simulink model "LRMate200Experimentor_Servo"  (R2015b)
settings: Solver=FixedStepDiscrete  StartTime=0.0  StopTime=10.0  FixedStep=si.tsv  RelTol=1e-3
model workspace (MATLAB code in the model file):
  | rsi = evalin('base', 'si.ri{1}');
undefined symbols (not defined in the file or in its folder): DiscIntNeverNeededParam, si
libraries: simulink x7
settings Model: ParameterArgumentNames=rsi  Creator=rluser  LastModifiedBy=Chin
settings SolverCC: EnableConcurrentExecution=on
settings DataIOCC: SaveFormat=Array
settings OptimizationCC: BlockReduction=off  OptimizeBlockIOStorage=off  BufferReuse=off  GlobalBufferReuse=off  ExpressionFolding=off  LocalBlockOutputs=off
settings DebuggingCC: SolverPrmCheckMsg=warning
settings HardwareCC: ProdBitPerPointer=32  ProdLargestAtomicFloat=None  ProdWordSize=32  ProdLongLongMode=on  ProdHWDeviceType=Generic->32-bit x86 compatible
settings RTWCC: SystemTargetFile=slrt.tlc  TemplateMakefile=slrt_default_tmf  Description=Simulink Real-Time  RTWCompilerOptimization=on
settings CodeAppCC: MaxIdLength=120
settings SimulinkRealTimeCC: GeneratePreprocessorConditionals=Disable all
settings ConfigComp: CovModelRefEnable=Off  CovSFcnEnable=off

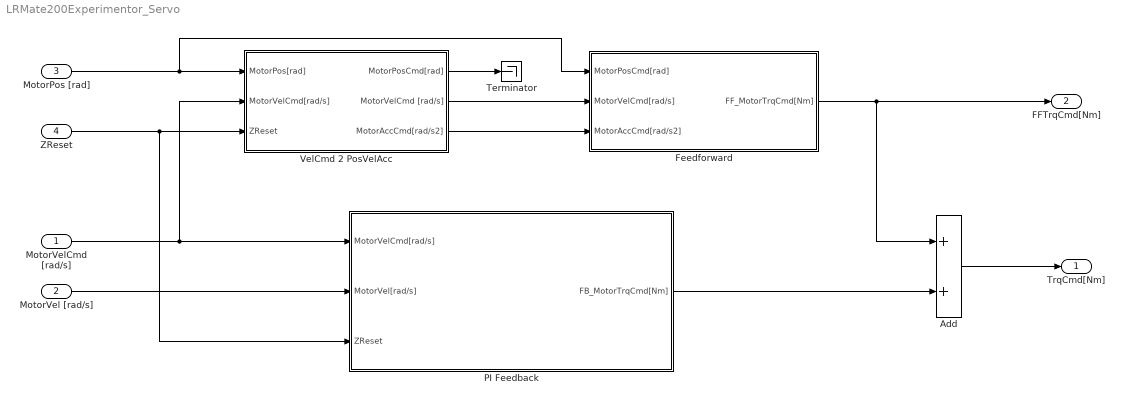
== system LRMate200Experimentor_Servo ==
  MotorVelCmd [rad/s] : Inport  PortDimensions=6
  MotorVel [rad/s] : Inport  Port=2  PortDimensions=6
  MotorPos [rad] : Inport  Port=3  PortDimensions=6
  ZReset : Inport  Port=4  OutDataTypeStr=boolean
  Add : Sum
  Feedforward : Subsystem
  PI Feedback : Subsystem
  Terminator : Terminator
  VelCmd 2 PosVelAcc : Subsystem
  TrqCmd[Nm] : Outport
  FFTrqCmd[Nm] : Outport  Port=2
  wires:
  MotorVel [rad/s]/1 -> PI Feedback/2(MotorVel[rad/s])
  MotorVelCmd [rad/s]/1 -> VelCmd 2 PosVelAcc/2(MotorVelCmd[rad/s]), PI Feedback/1(MotorVelCmd[rad/s])
  Add/1 -> TrqCmd[Nm]/1
  MotorPos [rad]/1 -> Feedforward/1(MotorPosCmd[rad]), VelCmd 2 PosVelAcc/1(MotorPos[rad])
  VelCmd 2 PosVelAcc/2(MotorVelCmd [rad/s]) -> Feedforward/2(MotorVelCmd[rad/s])
  VelCmd 2 PosVelAcc/3(MotorAccCmd[rad/s2]) -> Feedforward/3(MotorAccCmd[rad/s2])
  VelCmd 2 PosVelAcc/1(MotorPosCmd[rad]) -> Terminator/1
  ZReset/1 -> PI Feedback/3(ZReset), VelCmd 2 PosVelAcc/3(ZReset)
  PI Feedback/1(FB_MotorTrqCmd[Nm]) -> Add/2
  Feedforward/1(FF_MotorTrqCmd[Nm]) -> FFTrqCmd[Nm]/1, Add/1

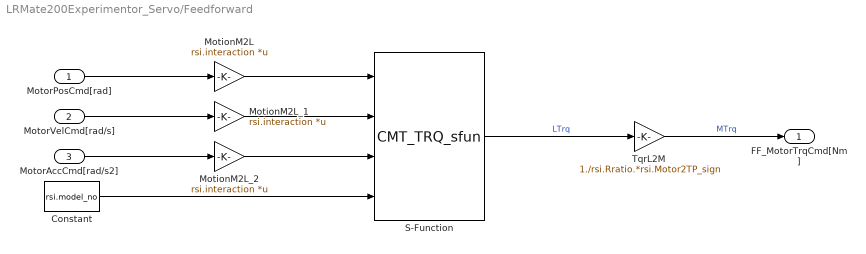
== system LRMate200Experimentor_Servo/Feedforward ==
  MotorPosCmd[rad] : Inport
  MotorVelCmd[rad/s] : Inport  Port=2
  MotorAccCmd[rad/s2] : Inport  Port=3
  Constant : Constant  Value=rsi.model_no
  MotionM2L : Gain  Gain=rsi.interaction  Multiplication=Matrix(K*u)
  MotionM2L_1 : Gain  Gain=rsi.interaction  Multiplication=Matrix(K*u)
  MotionM2L_2 : Gain  Gain=rsi.interaction  Multiplication=Matrix(K*u)
  S-Function : S-Function  FunctionName=CMT_TRQ_sfun  Parameters=si.tsv  SFunctionModules='CMT_TRQ'  SFunctionDeploymentMode=off  EnableBusSupport=off
  TqrL2M : Gain  Gain=1./rsi.Rratio.*rsi.Motor2TP_sign
  FF_MotorTrqCmd[Nm] : Outport
  wires:
  MotorPosCmd[rad]/1 -> MotionM2L/1
  MotorAccCmd[rad/s2]/1 -> MotionM2L_2/1
  MotionM2L/1 -> S-Function/1
  MotionM2L_1/1 -> S-Function/2
  MotionM2L_2/1 -> S-Function/3
  S-Function/1 -> TqrL2M/1  "LTrq"
  TqrL2M/1 -> FF_MotorTrqCmd[Nm]/1  "MTrq"
  MotorVelCmd[rad/s]/1 -> MotionM2L_1/1
  Constant/1 -> S-Function/4

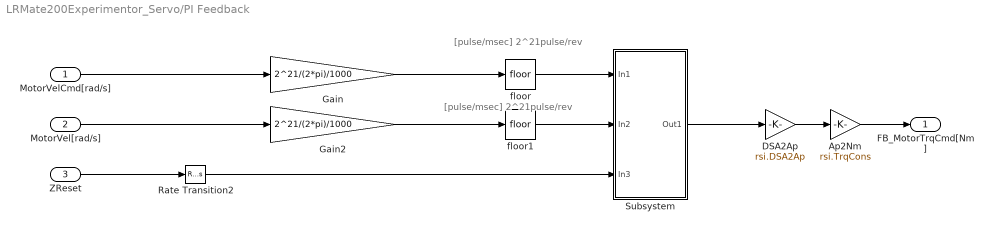
== system LRMate200Experimentor_Servo/PI Feedback ==
  note: [pulse/msec]
      | 2^21pulse/rev
  note: [pulse/msec]
      | 2^21pulse/rev
  MotorVelCmd[rad/s] : Inport
  MotorVel[rad/s] : Inport  Port=2
  ZReset : Inport  Port=3
  Ap2Nm : Gain  Gain=rsi.TrqCons
  DSA2Ap : Gain  Gain=rsi.DSA2Ap
  Gain : Gain  Gain=2^21/(2*pi)/1000  SaturateOnIntegerOverflow=on  OutDataTypeStr=Inherit: Same as input  ParamDataTypeStr=Inherit: Same as input
  Gain2 : Gain  Gain=2^21/(2*pi)/1000  SaturateOnIntegerOverflow=on  OutDataTypeStr=Inherit: Same as input  ParamDataTypeStr=Inherit: Same as input
  Rate Transition2 : RateTransition  OutPortSampleTime=si.tsv
  Subsystem : Subsystem
  floor : Rounding
  floor1 : Rounding
  FB_MotorTrqCmd[Nm] : Outport
  wires:
  ZReset/1 -> Rate Transition2/1
  Subsystem/1(Out1) -> DSA2Ap/1
  DSA2Ap/1 -> Ap2Nm/1
  Ap2Nm/1 -> FB_MotorTrqCmd[Nm]/1
  MotorVelCmd[rad/s]/1 -> Gain/1
  Gain/1 -> floor/1
  MotorVel[rad/s]/1 -> Gain2/1
  Gain2/1 -> floor1/1
  floor/1 -> Subsystem/1(In1)
  floor1/1 -> Subsystem/2(In2)
  Rate Transition2/1 -> Subsystem/3(In3)

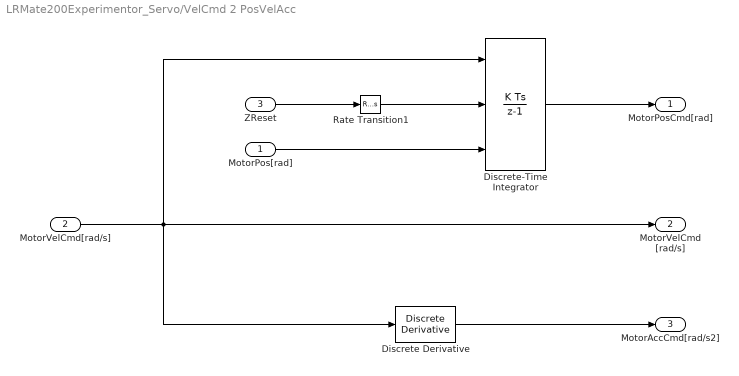
== system LRMate200Experimentor_Servo/VelCmd 2 PosVelAcc ==
  MotorPos[rad] : Inport
  MotorVelCmd[rad/s] : Inport  Port=2
  ZReset : Inport  Port=3
  Discrete Derivative : simulink/Discrete/Discrete Derivative  gainval=1.0  ICPrevScaledInput=0.0  InputProcessing=Inherited  OutMin=[]  OutMax=[]  OutDataType=fixdt(1, 16)  OutScaling=2^-10  DoSatur=off
  Discrete-Time Integrator : DiscreteIntegrator  ExternalReset=level  InitialConditionSource=external  InitialConditionSetting=State (most efficient)  SampleTime=si.tsv  ICPrevOutput=DiscIntNeverNeededParam  ICPrevScaledInput=DiscIntNeverNeededParam
  Rate Transition1 : RateTransition  OutPortSampleTime=si.tsv
  MotorPosCmd[rad] : Outport
  MotorVelCmd [rad/s] : Outport  Port=2
  MotorAccCmd[rad/s2] : Outport  Port=3
  wires:
  ZReset/1 -> Rate Transition1/1
  Rate Transition1/1 -> Discrete-Time Integrator/2
  Discrete-Time Integrator/1 -> MotorPosCmd[rad]/1
  Discrete Derivative/1 -> MotorAccCmd[rad/s2]/1
  MotorVelCmd[rad/s]/1 -> Discrete Derivative/1, Discrete-Time Integrator/1, MotorVelCmd [rad/s]/1
  MotorPos[rad]/1 -> Discrete-Time Integrator/3

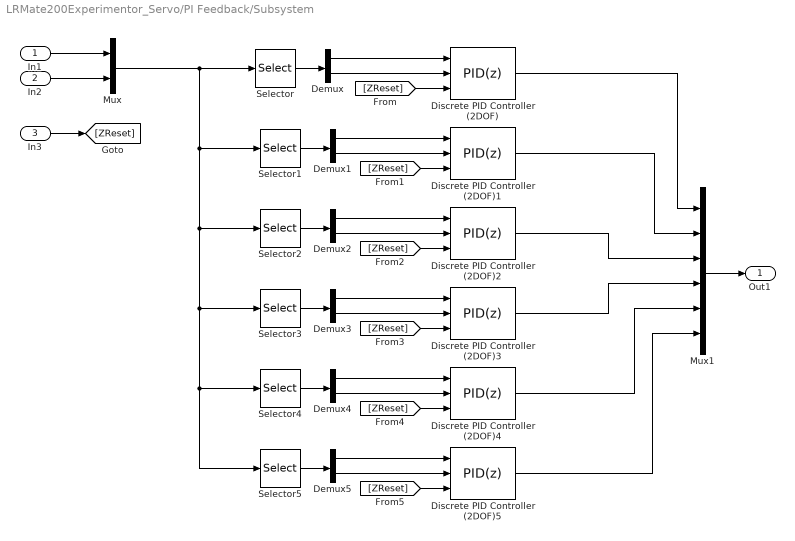
== system LRMate200Experimentor_Servo/PI Feedback/Subsystem ==
  In1 : Inport
  In2 : Inport  Port=2
  In3 : Inport  Port=3
  Demux{,1..5} (6 alike) : Demux  Outputs=2
  Discrete PID Controller (2DOF) : simulink/Continuous/PID Controller (2DOF)  Controller=PID  TimeDomain=Discrete-time  SampleTime=si.tsv  IntegratorMethod=Forward Euler  FilterMethod=Forward Euler  Form=Parallel  UseFilter=on  ControllerParametersSource=internal  P=rsi.kv(1)  I=rsi.ki(1)  D=0  N=100  b=1  c=1  InitialConditionSource=internal  InitialConditionForIntegrator=0  InitialConditionForFilter=0  ExternalReset=level  ZeroCross=off  LimitOutput=on  UpperSaturationLimit=3000  LowerSaturationLimit=-3000  LinearizeAsGain=off  AntiWindupMode=none  Kb=1  TrackingMode=off  Kt=1  PParamMin=[]  PParamMax=[]  IParamMin=[]  IParamMax=[]  DParamMin=[]  DParamMax=[]  NParamMin=[]  NParamMax=[]  bParamMin=[]  bParamMax=[]  cParamMin=[]  cParamMax=[]  KbParamMin=[]  KbParamMax=[]  KtParamMin=[]  KtParamMax=[]  POutMin=[]  POutMax=[]  IOutMin=[]  IOutMax=[]  DOutMin=[]  DOutMax=[]  NOutMin=[]  NOutMax=[]  bOutMin=[]  bOutMax=[]  cOutMin=[]  cOutMax=[]  KbOutMin=[]  KbOutMax=[]  KtOutMin=[]  KtOutMax=[]  IntegratorOutMin=[]  IntegratorOutMax=[]  FilterOutMin=[]  FilterOutMax=[]  SumOutMin=[]  SumOutMax=[]  Sum1OutMin=[]  Sum1OutMax=[]  Sum2OutMin=[]  Sum2OutMax=[]  Sum3OutMin=[]  Sum3OutMax=[]  SumI1OutMin=[]  SumI1OutMax=[]  SumI2OutMin=[]  SumI2OutMax=[]  SumI3OutMin=[]  SumI3OutMax=[]  SumDOutMin=[]  SumDOutMax=[]  SaturationOutMin=[]  SaturationOutMax=[]  IntegratorContinuousStateAttributes=''  IntegratorStateMustResolveToSignalObject=off  IntegratorRTWStateStorageClass=Auto  FilterContinuousStateAttributes=''  FilterStateMustResolveToSignalObject=off  FilterRTWStateStorageClass=Auto  DifferentiatorICPrevScaledInput=0  DifferentiatorOutMin=[]  DifferentiatorOutMax=[]
  Discrete PID Controller (2DOF)1 : simulink/Continuous/PID Controller (2DOF)  Controller=PID  TimeDomain=Discrete-time  SampleTime=si.tsv  IntegratorMethod=Forward Euler  FilterMethod=Forward Euler  Form=Parallel  UseFilter=on  ControllerParametersSource=internal  P=rsi.kv(2)  I=rsi.ki(2)  D=0  N=100  b=1  c=1  InitialConditionSource=internal  InitialConditionForIntegrator=0  InitialConditionForFilter=0  ExternalReset=level  ZeroCross=off  LimitOutput=on  UpperSaturationLimit=3000  LowerSaturationLimit=-3000  LinearizeAsGain=off  AntiWindupMode=none  Kb=1  TrackingMode=off  Kt=1  PParamMin=[]  PParamMax=[]  IParamMin=[]  IParamMax=[]  DParamMin=[]  DParamMax=[]  NParamMin=[]  NParamMax=[]  bParamMin=[]  bParamMax=[]  cParamMin=[]  cParamMax=[]  KbParamMin=[]  KbParamMax=[]  KtParamMin=[]  KtParamMax=[]  POutMin=[]  POutMax=[]  IOutMin=[]  IOutMax=[]  DOutMin=[]  DOutMax=[]  NOutMin=[]  NOutMax=[]  bOutMin=[]  bOutMax=[]  cOutMin=[]  cOutMax=[]  KbOutMin=[]  KbOutMax=[]  KtOutMin=[]  KtOutMax=[]  IntegratorOutMin=[]  IntegratorOutMax=[]  FilterOutMin=[]  FilterOutMax=[]  SumOutMin=[]  SumOutMax=[]  Sum1OutMin=[]  Sum1OutMax=[]  Sum2OutMin=[]  Sum2OutMax=[]  Sum3OutMin=[]  Sum3OutMax=[]  SumI1OutMin=[]  SumI1OutMax=[]  SumI2OutMin=[]  SumI2OutMax=[]  SumI3OutMin=[]  SumI3OutMax=[]  SumDOutMin=[]  SumDOutMax=[]  SaturationOutMin=[]  SaturationOutMax=[]  IntegratorContinuousStateAttributes=''  IntegratorStateMustResolveToSignalObject=off  IntegratorRTWStateStorageClass=Auto  FilterContinuousStateAttributes=''  FilterStateMustResolveToSignalObject=off  FilterRTWStateStorageClass=Auto  DifferentiatorICPrevScaledInput=0  DifferentiatorOutMin=[]  DifferentiatorOutMax=[]
  Discrete PID Controller (2DOF)2 : simulink/Continuous/PID Controller (2DOF)  Controller=PID  TimeDomain=Discrete-time  SampleTime=si.tsv  IntegratorMethod=Forward Euler  FilterMethod=Forward Euler  Form=Parallel  UseFilter=on  ControllerParametersSource=internal  P=rsi.kv(3)  I=rsi.ki(3)  D=0  N=100  b=1  c=1  InitialConditionSource=internal  InitialConditionForIntegrator=0  InitialConditionForFilter=0  ExternalReset=level  ZeroCross=off  LimitOutput=on  UpperSaturationLimit=3000  LowerSaturationLimit=-3000  LinearizeAsGain=off  AntiWindupMode=none  Kb=1  TrackingMode=off  Kt=1  PParamMin=[]  PParamMax=[]  IParamMin=[]  IParamMax=[]  DParamMin=[]  DParamMax=[]  NParamMin=[]  NParamMax=[]  bParamMin=[]  bParamMax=[]  cParamMin=[]  cParamMax=[]  KbParamMin=[]  KbParamMax=[]  KtParamMin=[]  KtParamMax=[]  POutMin=[]  POutMax=[]  IOutMin=[]  IOutMax=[]  DOutMin=[]  DOutMax=[]  NOutMin=[]  NOutMax=[]  bOutMin=[]  bOutMax=[]  cOutMin=[]  cOutMax=[]  KbOutMin=[]  KbOutMax=[]  KtOutMin=[]  KtOutMax=[]  IntegratorOutMin=[]  IntegratorOutMax=[]  FilterOutMin=[]  FilterOutMax=[]  SumOutMin=[]  SumOutMax=[]  Sum1OutMin=[]  Sum1OutMax=[]  Sum2OutMin=[]  Sum2OutMax=[]  Sum3OutMin=[]  Sum3OutMax=[]  SumI1OutMin=[]  SumI1OutMax=[]  SumI2OutMin=[]  SumI2OutMax=[]  SumI3OutMin=[]  SumI3OutMax=[]  SumDOutMin=[]  SumDOutMax=[]  SaturationOutMin=[]  SaturationOutMax=[]  IntegratorContinuousStateAttributes=''  IntegratorStateMustResolveToSignalObject=off  IntegratorRTWStateStorageClass=Auto  FilterContinuousStateAttributes=''  FilterStateMustResolveToSignalObject=off  FilterRTWStateStorageClass=Auto  DifferentiatorICPrevScaledInput=0  DifferentiatorOutMin=[]  DifferentiatorOutMax=[]
  Discrete PID Controller (2DOF)3 : simulink/Continuous/PID Controller (2DOF)  Controller=PID  TimeDomain=Discrete-time  SampleTime=si.tsv  IntegratorMethod=Forward Euler  FilterMethod=Forward Euler  Form=Parallel  UseFilter=on  ControllerParametersSource=internal  P=rsi.kv(4)  I=rsi.ki(4)  D=0  N=100  b=1  c=1  InitialConditionSource=internal  InitialConditionForIntegrator=0  InitialConditionForFilter=0  ExternalReset=level  ZeroCross=off  LimitOutput=on  UpperSaturationLimit=3000  LowerSaturationLimit=-3000  LinearizeAsGain=off  AntiWindupMode=none  Kb=1  TrackingMode=off  Kt=1  PParamMin=[]  PParamMax=[]  IParamMin=[]  IParamMax=[]  DParamMin=[]  DParamMax=[]  NParamMin=[]  NParamMax=[]  bParamMin=[]  bParamMax=[]  cParamMin=[]  cParamMax=[]  KbParamMin=[]  KbParamMax=[]  KtParamMin=[]  KtParamMax=[]  POutMin=[]  POutMax=[]  IOutMin=[]  IOutMax=[]  DOutMin=[]  DOutMax=[]  NOutMin=[]  NOutMax=[]  bOutMin=[]  bOutMax=[]  cOutMin=[]  cOutMax=[]  KbOutMin=[]  KbOutMax=[]  KtOutMin=[]  KtOutMax=[]  IntegratorOutMin=[]  IntegratorOutMax=[]  FilterOutMin=[]  FilterOutMax=[]  SumOutMin=[]  SumOutMax=[]  Sum1OutMin=[]  Sum1OutMax=[]  Sum2OutMin=[]  Sum2OutMax=[]  Sum3OutMin=[]  Sum3OutMax=[]  SumI1OutMin=[]  SumI1OutMax=[]  SumI2OutMin=[]  SumI2OutMax=[]  SumI3OutMin=[]  SumI3OutMax=[]  SumDOutMin=[]  SumDOutMax=[]  SaturationOutMin=[]  SaturationOutMax=[]  IntegratorContinuousStateAttributes=''  IntegratorStateMustResolveToSignalObject=off  IntegratorRTWStateStorageClass=Auto  FilterContinuousStateAttributes=''  FilterStateMustResolveToSignalObject=off  FilterRTWStateStorageClass=Auto  DifferentiatorICPrevScaledInput=0  DifferentiatorOutMin=[]  DifferentiatorOutMax=[]
  Discrete PID Controller (2DOF)4 : simulink/Continuous/PID Controller (2DOF)  Controller=PID  TimeDomain=Discrete-time  SampleTime=si.tsv  IntegratorMethod=Forward Euler  FilterMethod=Forward Euler  Form=Parallel  UseFilter=on  ControllerParametersSource=internal  P=rsi.kv(5)  I=rsi.ki(5)  D=0  N=100  b=1  c=1  InitialConditionSource=internal  InitialConditionForIntegrator=0  InitialConditionForFilter=0  ExternalReset=level  ZeroCross=off  LimitOutput=on  UpperSaturationLimit=3000  LowerSaturationLimit=-3000  LinearizeAsGain=off  AntiWindupMode=none  Kb=1  TrackingMode=off  Kt=1  PParamMin=[]  PParamMax=[]  IParamMin=[]  IParamMax=[]  DParamMin=[]  DParamMax=[]  NParamMin=[]  NParamMax=[]  bParamMin=[]  bParamMax=[]  cParamMin=[]  cParamMax=[]  KbParamMin=[]  KbParamMax=[]  KtParamMin=[]  KtParamMax=[]  POutMin=[]  POutMax=[]  IOutMin=[]  IOutMax=[]  DOutMin=[]  DOutMax=[]  NOutMin=[]  NOutMax=[]  bOutMin=[]  bOutMax=[]  cOutMin=[]  cOutMax=[]  KbOutMin=[]  KbOutMax=[]  KtOutMin=[]  KtOutMax=[]  IntegratorOutMin=[]  IntegratorOutMax=[]  FilterOutMin=[]  FilterOutMax=[]  SumOutMin=[]  SumOutMax=[]  Sum1OutMin=[]  Sum1OutMax=[]  Sum2OutMin=[]  Sum2OutMax=[]  Sum3OutMin=[]  Sum3OutMax=[]  SumI1OutMin=[]  SumI1OutMax=[]  SumI2OutMin=[]  SumI2OutMax=[]  SumI3OutMin=[]  SumI3OutMax=[]  SumDOutMin=[]  SumDOutMax=[]  SaturationOutMin=[]  SaturationOutMax=[]  IntegratorContinuousStateAttributes=''  IntegratorStateMustResolveToSignalObject=off  IntegratorRTWStateStorageClass=Auto  FilterContinuousStateAttributes=''  FilterStateMustResolveToSignalObject=off  FilterRTWStateStorageClass=Auto  DifferentiatorICPrevScaledInput=0  DifferentiatorOutMin=[]  DifferentiatorOutMax=[]
  Discrete PID Controller (2DOF)5 : simulink/Continuous/PID Controller (2DOF)  Controller=PID  TimeDomain=Discrete-time  SampleTime=si.tsv  IntegratorMethod=Forward Euler  FilterMethod=Forward Euler  Form=Parallel  UseFilter=on  ControllerParametersSource=internal  P=rsi.kv(6)  I=rsi.ki(6)  D=0  N=100  b=1  c=1  InitialConditionSource=internal  InitialConditionForIntegrator=0  InitialConditionForFilter=0  ExternalReset=level  ZeroCross=off  LimitOutput=on  UpperSaturationLimit=3000  LowerSaturationLimit=-3000  LinearizeAsGain=off  AntiWindupMode=none  Kb=1  TrackingMode=off  Kt=1  PParamMin=[]  PParamMax=[]  IParamMin=[]  IParamMax=[]  DParamMin=[]  DParamMax=[]  NParamMin=[]  NParamMax=[]  bParamMin=[]  bParamMax=[]  cParamMin=[]  cParamMax=[]  KbParamMin=[]  KbParamMax=[]  KtParamMin=[]  KtParamMax=[]  POutMin=[]  POutMax=[]  IOutMin=[]  IOutMax=[]  DOutMin=[]  DOutMax=[]  NOutMin=[]  NOutMax=[]  bOutMin=[]  bOutMax=[]  cOutMin=[]  cOutMax=[]  KbOutMin=[]  KbOutMax=[]  KtOutMin=[]  KtOutMax=[]  IntegratorOutMin=[]  IntegratorOutMax=[]  FilterOutMin=[]  FilterOutMax=[]  SumOutMin=[]  SumOutMax=[]  Sum1OutMin=[]  Sum1OutMax=[]  Sum2OutMin=[]  Sum2OutMax=[]  Sum3OutMin=[]  Sum3OutMax=[]  SumI1OutMin=[]  SumI1OutMax=[]  SumI2OutMin=[]  SumI2OutMax=[]  SumI3OutMin=[]  SumI3OutMax=[]  SumDOutMin=[]  SumDOutMax=[]  SaturationOutMin=[]  SaturationOutMax=[]  IntegratorContinuousStateAttributes=''  IntegratorStateMustResolveToSignalObject=off  IntegratorRTWStateStorageClass=Auto  FilterContinuousStateAttributes=''  FilterStateMustResolveToSignalObject=off  FilterRTWStateStorageClass=Auto  DifferentiatorICPrevScaledInput=0  DifferentiatorOutMin=[]  DifferentiatorOutMax=[]
  Mux : Mux  Inputs=2
  Mux1 : Mux  Inputs=6
  Selector : Selector  InputPortWidth=12  IndexOptions=Index vector (dialog)  Indices=[1 7]  OutputSizes=1
  Selector1 : Selector  InputPortWidth=12  IndexOptions=Index vector (dialog)  Indices=[2 8]  OutputSizes=1
  Selector2 : Selector  InputPortWidth=12  IndexOptions=Index vector (dialog)  Indices=[3 9]  OutputSizes=1
  Selector3 : Selector  InputPortWidth=12  IndexOptions=Index vector (dialog)  Indices=[4 10]  OutputSizes=1
  Selector4 : Selector  InputPortWidth=12  IndexOptions=Index vector (dialog)  Indices=[5 11]  OutputSizes=1
  Selector5 : Selector  InputPortWidth=12  IndexOptions=Index vector (dialog)  Indices=[6 12]  OutputSizes=1
  Out1 : Outport
  wires:
  In1/1 -> Mux/1
  In2/1 -> Mux/2
  Selector/1 -> Demux/1
  Demux/1 -> Discrete PID Controller (2DOF)/1
  Demux/2 -> Discrete PID Controller (2DOF)/2
  In3/1 -> [ZReset]
  [ZReset] -> Discrete PID Controller (2DOF)/3
  Selector1/1 -> Demux1/1
  Demux1/1 -> Discrete PID Controller (2DOF)1/1
  Demux1/2 -> Discrete PID Controller (2DOF)1/2
  [ZReset] -> Discrete PID Controller (2DOF)1/3
  Selector2/1 -> Demux2/1
  Demux2/1 -> Discrete PID Controller (2DOF)2/1
  Demux2/2 -> Discrete PID Controller (2DOF)2/2
  [ZReset] -> Discrete PID Controller (2DOF)2/3
  Selector3/1 -> Demux3/1
  Demux3/1 -> Discrete PID Controller (2DOF)3/1
  Demux3/2 -> Discrete PID Controller (2DOF)3/2
  [ZReset] -> Discrete PID Controller (2DOF)3/3
  Selector4/1 -> Demux4/1
  Demux4/1 -> Discrete PID Controller (2DOF)4/1
  Demux4/2 -> Discrete PID Controller (2DOF)4/2
  [ZReset] -> Discrete PID Controller (2DOF)4/3
  Mux/1 -> Selector1/1, Selector4/1, Selector5/1, Selector3/1, Selector2/1, Selector/1
  Selector5/1 -> Demux5/1
  Demux5/1 -> Discrete PID Controller (2DOF)5/1
  Demux5/2 -> Discrete PID Controller (2DOF)5/2
  [ZReset] -> Discrete PID Controller (2DOF)5/3
  Discrete PID Controller (2DOF)/1 -> Mux1/1
  Discrete PID Controller (2DOF)1/1 -> Mux1/2
  Discrete PID Controller (2DOF)2/1 -> Mux1/3
  Discrete PID Controller (2DOF)3/1 -> Mux1/4
  Discrete PID Controller (2DOF)4/1 -> Mux1/5
  Discrete PID Controller (2DOF)5/1 -> Mux1/6
  Mux1/1 -> Out1/1
